simulink model "imageprocessing"  (R2024a)
settings: Solver=VariableStepAuto  StartTime=0.0  StopTime=10.0  RelTol=1e-3
undefined symbols (not defined in the file): CIRCLE_PTS, gray, ZEROS
libraries: visiontextngfix x1, parrotlib x1, simulink x1
settings Model: Creator=tejas  LastModifiedBy=tejas

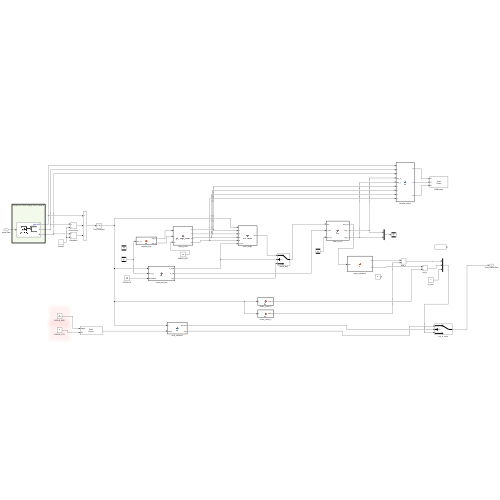
[thumbnail: Simulink's stored preview of the top-level diagram]
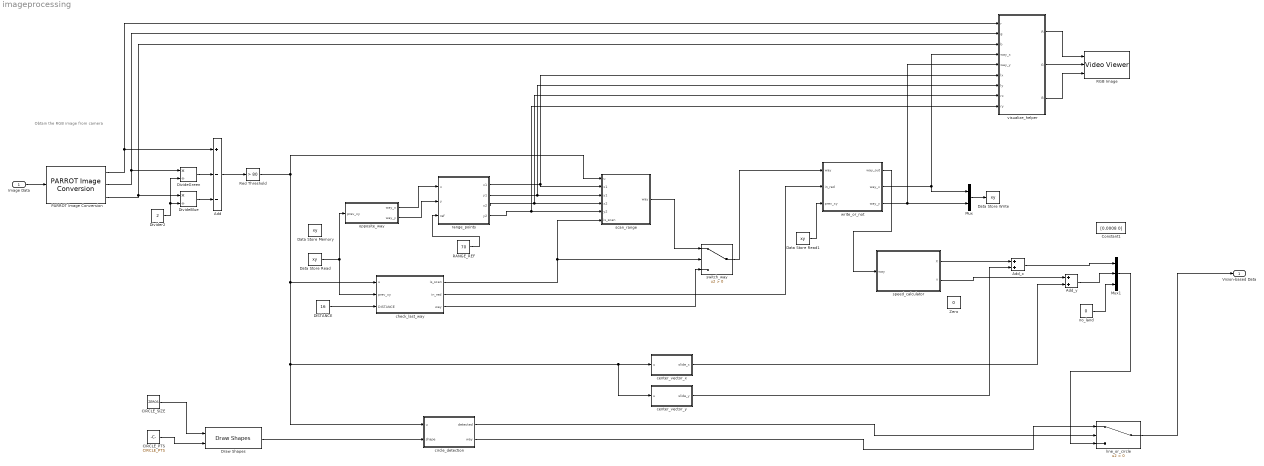
== system imageprocessing ==
  note: Obtain the RGB image from camera
  Image Data : Inport
  Add : Sum  Inputs=+--
  Add_x : Sum
  Add_y : Sum
  CIRCLE_PTS : Constant  Value=CIRCLE_PTS
  CIRCLE_SIZE : Constant  Value=ZEROS
  Constant1 : Constant  Value=[0.0008 0]
  DISTANCE : Constant  Value=16
  Data Store Memory : DataStoreMemory  DataStoreName=xy  ReadBeforeWriteMsg=warning  WriteAfterWriteMsg=warning  WriteAfterReadMsg=warning  InitialValue=[0 0]  ShowAdditionalParam=off
  Data Store Read : DataStoreRead  DataStoreName=xy  IndexOptions=Index vector (dialog)  Indices=1  OutputSizes=1
  Data Store Read1 : DataStoreRead  DataStoreName=xy  IndexOptions=Index vector (dialog)  Indices=1  OutputSizes=1
  Data Store Write : DataStoreWrite  DataStoreName=xy  IndexOptions=Index vector (dialog)  Indices=1  OutputSizes=1
  DivideBlue : Product  Inputs=*/
  DivideGreen : Product  Inputs=*/
  Divider2 : Constant  Value=2
  Draw Shapes : visiontextngfix/Draw Shapes  shape=Circles  fill=on  lineWidth=1  fillClrSource=Specify via dialog  display=White  intensity=200  color=[200 255 100]  opacity=1  viewport=Entire image  antialiasing=off  inType=Obsolete  imagePorts=One multidimensional signal  roundingMode=Floor  overflowMode=off  memoryMode=Specify word length  memoryWordLength=16  prodOutputMode=Binary point scaling  prodOutputWordLength=32  prodOutputFracLength=14  memoryFracLength=15
  Mux : Mux  Inputs=2
  Mux1 : Mux  Inputs=3
  PARROT Image Conversion : parrotlib/PARROT Image Conversion  ImageFormat=RGB  R=on  Y=on  G=on  U=on  B=on  V=on
  RANGE_REF : Constant  Value=70
  RGB Image : VideoViewer  imagePorts=separate color signals  colormapValue=gray(256)  FigPos=[2703.4 754 730.4 526.4]
  Red Threshold : simulink/Logic and Bit Operations/Compare To Constant  relop=>  const=80  OutDataTypeStr=boolean
  Zero : Constant  Value=0  OutDataTypeStr=Inherit: Inherit via back propagation
  center_vector_x : MATLAB Function  TreatAsAtomicUnit=on
  center_vector_y : MATLAB Function  TreatAsAtomicUnit=on
  check_last_way : MATLAB Function  TreatAsAtomicUnit=on
  circle_detection : MATLAB Function  TreatAsAtomicUnit=on
  line_or_circle : Switch  Criteria=u2 > Threshold  SaturateOnIntegerOverflow=off  InputSameDT=off
  no_land : Constant  Value=0
  opposite_way : MATLAB Function  TreatAsAtomicUnit=on
  range_points : MATLAB Function  TreatAsAtomicUnit=on
  scan_range : MATLAB Function  TreatAsAtomicUnit=on
  speed_calculator : MATLAB Function  TreatAsAtomicUnit=on
  switch_way : Switch  Criteria=u2 > Threshold  SaturateOnIntegerOverflow=off  InputSameDT=off
  visualize_helper : MATLAB Function  TreatAsAtomicUnit=on
  write_or_not : MATLAB Function  TreatAsAtomicUnit=on
  Vision-based Data : Outport  VectorParamsAs1DForOutWhenUnconnected=off
  wires:
  write_or_not/3(way_y) -> Mux/2, visualize_helper/5(way_y)
  write_or_not/2(way_x) -> Mux/1, visualize_helper/4(way_x)
  range_points/4(y2) -> scan_range/5(y2), visualize_helper/9(ry)
  speed_calculator/2(Y) -> Add_y/1
  opposite_way/2(way_y) -> range_points/2(y)
  visualize_helper/2(G) -> RGB Image/2
  Mux/1 -> Data Store Write/1
  PARROT Image Conversion/1 -> Add/1, visualize_helper/1(r)
  Image Data/1 -> PARROT Image Conversion/1
  range_points/1(x1) -> scan_range/2(x1), visualize_helper/6(lx)
  PARROT Image Conversion/3 -> visualize_helper/3(b), DivideBlue/1
  RANGE_REF/1 -> range_points/3(ref)
  write_or_not/1(way_out) -> speed_calculator/1(way)
  check_last_way/2(in_red) -> write_or_not/2(in_red)
  Data Store Read1/1 -> write_or_not/3(prev_xy)
  visualize_helper/1(R) -> RGB Image/1
  no_land/1 -> Mux1/3
  CIRCLE_PTS/1 -> Draw Shapes/2
  circle_detection/1(detected) -> line_or_circle/2
  DivideBlue/1 -> Add/3
  Data Store Read/1 -> opposite_way/1(prev_xy), check_last_way/2(prev_xy)
  center_vector_x/1(slide_x) -> Add_y/2
  PARROT Image Conversion/2 -> DivideGreen/1, visualize_helper/2(g)
  CIRCLE_SIZE/1 -> Draw Shapes/1
  check_last_way/1(is_scan) -> scan_range/6(is_scan), switch_way/2
  Add_x/1 -> Mux1/1
  circle_detection/2(way) -> line_or_circle/1
  speed_calculator/1(X) -> Add_x/1
  check_last_way/3(way) -> switch_way/3
  Add/1 -> Red Threshold/1
  range_points/3(x2) -> scan_range/4(x2), visualize_helper/8(rx)
  Divider2/1 -> DivideGreen/2, DivideBlue/2
  Red Threshold/1 -> circle_detection/1(u), center_vector_x/1(u), center_vector_y/1(u), check_last_way/1(u), scan_range/1(u)
  DivideGreen/1 -> Add/2
  switch_way/1 -> write_or_not/1(way)
  center_vector_y/1(slide_y) -> Add_x/2
  Add_y/1 -> Mux1/2
  opposite_way/1(way_x) -> range_points/1(x)
  scan_range/1(way) -> switch_way/1
  line_or_circle/1 -> Vision-based Data/1
  DISTANCE/1 -> check_last_way/3(DISTANCE)
  Mux1/1 -> line_or_circle/3
  Draw Shapes/1 -> circle_detection/2(shape)
  range_points/2(y1) -> scan_range/3(y1), visualize_helper/7(ly)
  visualize_helper/3(B) -> RGB Image/3

== matlab function imageprocessing/write_or_not ==
  data: way input; way_out output; in_red input; prev_xy input; way_x output; way_y output
function [way_out, way_x, way_y] = fcn(way, in_red, prev_xy)

x = way(1);
y = way(2);
speed = way(3);

if in_red
    X = x;   Y = y;
    way_x = x;  way_y = y;
else
    X = x;  Y = y; 
    way_x = prev_xy(1);  
    way_y = prev_xy(2);
end

way_out = [X Y speed];

%fprintf('X = %f | Y = %f\n', way_x, way_y);
end

== matlab function imageprocessing/speed_calculator ==
  data: way input; X output; Y output
function [X,Y] = fcn(way)

x = way(1);
y = way(2);
speed = way(3);

if speed == 100
    speed = 200;
elseif speed < 60
    speed = 60;
end


X = (60-x) / 10000000 * speed;
Y = (y-80) / 10000000 * speed;


%fprintf(' --- speed: %f | ', speed); fprintf('vectors: X=%.5f | Y=%.5f\n', X, Y);

end

== matlab function imageprocessing/opposite_way ==
  data: way_x output; prev_xy input; way_y output
function [way_x, way_y] = fcn(prev_xy)

    x = prev_xy(1);
    y = prev_xy(2);
    
    if x == 0 || y == 0
        way_x = 0;
        way_y = 0;
    else
        way_x = 60 + (60 - x) + 1;
        way_y = 80 + (80 - y) + 1;
    end

    %fprintf('opposite: %.0f %.0f -> %.0f %.0f\n', x, y, way_x, way_y);
end

== matlab function imageprocessing/center_vector_x ==
  data: u input; slide_x output
function slide_x = fcn(u)
c1 = 60; 
c2 = 80;
left_p = 0;
right_p = 0;
middle_point = u(c1, c2);
compare = ~middle_point;
for i = c2:-1:60 % <---  look left
    if u(c1, i) == compare
        left_p = i;
        break
    end
end
for i = c2:100 % --->   look right
    if u(c1, i) == compare
        right_p = i;
        break
    end
end

slide_x = 0;
if left_p ~= 0 && right_p ~= 0 % in line
    if middle_point == 1
        vr = right_p - c2;  % length right 
        vl = c2 - left_p;   % length left
        diff = vr-vl;
        slide_x = get_speed(diff) * 20;
    end
end
end

function T = get_speed(t)

if t > 0
    if t < 1
        T = 0.000001;
    elseif t < 5
        T = 0.000002;
    elseif t < 10
        T = 0.000003;
    elseif t < 15
        T = 0.000004;
    elseif t < 20
        T = 0.000005;
    else
        T = 0.000006;
    end
else
    if t < -20
        T = -0.000006;
    elseif t < -15
        T = -0.000005;
    elseif t < -10
        T = -0.000004;
    elseif t < -5
        T = -0.000003;
    elseif t < -1
        T = -0.000002;
    else
        T = -0.000001;
    end
end

end

== matlab function imageprocessing/range_points ==
  data: x input; x1 output; y input; ref input; y1 output; x2 output; y2 output
function [x1,y1, x2,y2] = get_range_points(x,y, ref)

% x1, y1 are left
% x2, y2 are right 
% according to center-to-edge vector.

W = edge_number(x,y);

if W == 1
    y1 = y - ref;
    if y1 < 1
        x1 = x - y1;
        y1 = 1;
    else
        x1 = x;
    end

    y2 = y + ref;
    if y2 > 160
        x2 = y2-160;
        y2 = 160;
    else
        x2 = x;
    end
elseif W == 2
    x1 = x + ref;
    if x1 > 120
        y1 = x1 - 120;
        x1 = 120;
    else
        y1 = y;
    end

    x2 = x - ref;
    if x2 < 1
        y2 = abs(x2) + 1;
        x2 = 1;
    else
        y2 = y;
    end
elseif W == 4
    x1 = x - ref;
    if x1 < 1
        y1 = 160 + x1;
        x1 = 1;
    else
        y1 = 160;
    end

    x2 = x + ref;
    if x2 > 120
        y2 = 160 - (x2 - 120);
        x2 = 120;
    else
        y2 = y;
    end
elseif W == 3
    y1 = y + ref;
    if y1 > 160
        x1 = 120 - (y1-160);
        y1 = 160;
    else
        x1 = x;
    end

    y2 = y - ref;
    if y2 < 1
        x2 = 120 + y2;
        y2 = 1;
    else
        x2 = x;
    end
else
    x1 = 1; y1 = 1;
    x2 = 1; y2 = 2;
end

%fprintf('range_points: %.0f-%.0f  to  %.0f-%.0f\n', x1,y1, x2,y2);

end

== matlab function imageprocessing/center_vector_y ==
  data: u input; slide_y output
function slide_y = fcn(u)
c1 = 60; 
c2 = 80;
up_p = 0;
down_p = 0;
middle_point = u(c1,c2);
compare = ~middle_point;
for i = c1:-1:40 % look up
    if u(i, c2) == compare
        up_p = i;
        break
    end
end
for i = c1:80 % look down
    if u(i, c2) == compare
        down_p = i;
        break
    end
end
slide_y = 0;
if up_p ~= 0 && down_p ~= 0  % in line
    if middle_point == 1
        vu = down_p - c1;  %length up
        vd = c1 - up_p;    %length down
        diff = vd-vu;
        
        slide_y = get_speed(diff) * 20;
    end
end

end
function T = get_speed(t)

if t > 0
    if t <= 1
        T = 0.000001;
    elseif t < 5
        T = 0.000002;
    elseif t < 10
        T = 0.000003;
    elseif t < 15
        T = 0.000005;
    elseif t < 20
        T = 0.000005;
    else
        T = 0.000005;
    end
else
    if t < -20
        T = -0.000005;
    elseif t < -15
        T = -0.000005;
    elseif t < -10
        T = -0.000004;
    elseif t <= -5
        T = -0.000003;
    elseif t < -1
        T = -0.000002;
    else
        T = -0.000001;
    end
end
end

== matlab function imageprocessing/scan_range ==
  data: way output; u input; x1 input; y1 input; x2 input; y2 input; is_scan input
function way  = scan_range(u, x1,y1, x2,y2, is_scan)

way_x = 1;
way_y = 2;
speed = 0;
in_red_line = u(60, 80);


persistent prev_endless_x;
persistent prev_endless_y;

if is_scan
    if in_red_line == 1  % ------ inside red-line ------
    
        t = 0;
        mx = 0;

        mx_endless_x = [0 0];
        mx_endless_y = [0 0];
        mx_t = [0 0];

        last_endless = false;
        index_of_endless = 0;
        
        w1 = edge_number(x1,y1);
        xi = x1;  yi = y1; k = 1;
        
        if w1 == 1 || w1 == 4
            k = -1;
        end
        
        
        while xi ~= x2 || yi ~= y2
            returned = line_drawer(60, 80, xi, yi, u, 0);

            if returned == 0 % if endless

                if last_endless == false
                    last_endless = true;
                    index_of_endless = index_of_endless + 1;
                end
                if index_of_endless > 2
                    break;
                end
                
                mx_endless_x(index_of_endless) = mx_endless_x(index_of_endless) + xi;
                mx_endless_y(index_of_endless) = mx_endless_y(index_of_endless) + yi;
                mx_t(index_of_endless) = mx_t(index_of_endless) + 1;

            else
                last_endless = false;
                if returned > mx
                    mx = returned;
                    way_x = xi; 
                    way_y = yi;
                    t = 1;
                end
            end

            % İteration
            temp_w = edge_number(xi, yi);
            if temp_w == 1 || temp_w == 3
                yi = yi + k;
            else
                xi = xi + k;
            end
            if xi < 1
                yi = 159; xi = 1; k = -1;
            elseif xi > 120
                xi = 120; yi = 2; k = 1;
            elseif yi < 1
                yi = 1; xi = 2; k = 1;
            elseif yi > 160
                yi = 160; xi = 119; k = -1;
            end
        end % while end


        if index_of_endless == 1 % ---------- 1 endless ------------
            %fprintf('only one endless!\n');
            way_x = mx_endless_x(1);
            way_y = mx_endless_y(1);
            t = mx_t(1);

            way_x = round(way_x/t);
            way_y = round(way_y/t);
            [way_x, way_y] = nearest_edge(way_x, way_y);

            prev_endless_x = 60 + (60 - way_x) + 1;
            prev_endless_y = 80 + (80 - way_y) + 1;

        elseif index_of_endless == 2 % ---------- 2 endless ------------
            
            if isempty(prev_endless_x)
                way_x = mx_endless_x(1);
                way_y = mx_endless_y(1);
                t = mx_t(1);
    
                way_x = round(way_x/t);
                way_y = round(way_y/t);
                [way_x, way_y] = nearest_edge(way_x, way_y);
    
                prev_endless_x = 60 + (60 - way_x) + 1;
                prev_endless_y = 80 + (80 - way_y) + 1;
            else
                mid_calculated = [0 0; 0 0];
                for i = 1:2
                    x = mx_endless_x(i);
                    y = mx_endless_y(i);
                    t = mx_t(i);

                    x = round(x/t);
                    y = round(y/t);
                    
                    [x,y] = nearest_edge(x, y);
                    
                    mid_calculated(i, 1) = x;
                    mid_calculated(i, 2) = y;
                end
                %fprintf('calculated = %.0f %.0f  | %.0f %.0f\n', ...
                %    mid_calculated(1,1), mid_calculated(1,2), ...
                %    mid_calculated(2,1), mid_calculated(2,2));

                diff_x1 = prev_endless_x-mid_calculated(1,1);
                diff_y1 = prev_endless_y-mid_calculated(1,2);
                diff_x2 = prev_endless_x-mid_calculated(2,1);
                diff_y2 = prev_endless_y-mid_calculated(2,2);
                diff1 = sqrt(diff_x1*diff_x1 + diff_y1*diff_y1);
                diff2 = sqrt(diff_x2*diff_x2 + diff_y2*diff_y2);

                if diff1 > diff2
                    way_x = mid_calculated(1,1);
                    way_y = mid_calculated(1,2);
                else
                    way_x = mid_calculated(2,1);
                    way_y = mid_calculated(2,2);
                end
                
                prev_endless_x = 60 + (60 - way_x) + 1;
                prev_endless_y = 80 + (80 - way_y) + 1;
                
            end
        else % ---------- NO endless ------------
            speed = mx;
        end

        

    else % ----------------- outside red line ----------------------
        x1 = 2; y1 = 1;
        x2 = 1; y2 = 1;
        
        ENDLESS = 100;
        mn = ENDLESS;
        w1 = edge_number(x1,y1);
        xi = x1;  yi = y1;  k = 1;
        if w1 == 1 || w1 == 4
            k = -1;
        end
        
        while xi ~= x2 || yi ~= y2
            returned = line_drawer(60, 80, xi, yi, u, 1);
    
            if returned > 0 && returned < mn
                mn = returned;
                way_x = xi;
                way_y = yi;
            end
    
            % İteration
            temp_w = edge_number(xi, yi);
            if temp_w == 1 || temp_w == 3
                yi = yi + k;
            else
                xi = xi + k;
            end
            if xi < 1
                yi = 159; xi = 1; k = -1;
            elseif xi > 120
                xi = 120; yi = 2; k = 1;
            elseif yi < 1
                yi = 1; xi = 2; k = 1;
            elseif yi > 160
                yi = 160; xi = 119; k = -1;
            end
        end % while
        
        speed = 100;
        if mn < 60
            speed = 60;
        end
    end % if redline end

end % is_scan

way = [way_x, way_y, speed];

end % function end

== matlab function imageprocessing/check_last_way ==
  data: u input; is_scan output; in_red output; prev_xy input; DISTANCE input; way output
function [is_scan, in_red, way]  = fcn(u, prev_xy, DISTANCE)

prev_x = prev_xy(1);
prev_y = prev_xy(2);

in_red = u(60, 80);
compare = ~in_red;

is_scan = 0;
way_x = 1;
way_y = 1;
speed = 0;

if prev_x == 0 || prev_y == 0
    is_scan = 1;
else 
    if u(prev_x, prev_y) == 1 

        % endless continue ------------------------------
        [ref_x, ref_y] = middle_point_of_endless_line(u, prev_x, prev_y);

        way_x = prev_x + ref_x;
        way_y = prev_y + ref_y;
        
        if way_y > 160
            if way_x == 120 
                way_x = 120 - mod(way_y, 160);
            elseif way_x == 1 
                way_x = mod(way_y, 160);
            end
            way_y = 160;
            
        elseif way_y < 1
            if way_x == 120 
                way_x = 120 - abs(way_y);
            elseif way_x == 1 
                way_x = abs(way_y); 
            end
            way_y = 1;
            
        elseif way_x < 1
            if way_y == 160
                way_y = 160 - abs(way_x);
            elseif way_y == 1
                way_y = abs(way_x);
            end
            way_x = 1;
            
        elseif way_x > 120
            if way_y == 160
                way_y = 160 - (way_x - 120);
            elseif way_y == 1
                way_y = way_x - 120;
            end
            way_x = 120;
        end

        %{
        if way_x < 1   way_x = 1;   end
        if way_x > 120 way_x = 120; end
        if way_y < 1   way_y = 1;   end
        if way_y > 160 way_y = 160; end
        %}
        speed = 100;

    else 
        
        % endless dissappeared ----------------------------
        if in_red
            distance = line_drawer(60, 80, prev_x, prev_y, u, compare);
            if distance < DISTANCE
                is_scan = 1;
                speed = 0;
            else
                speed = distance;
            end
            
            way_x = prev_x;
            way_y = prev_y;
        else
            is_scan = 1;
            way_x = prev_x;
            way_y = prev_y;
            speed = 40;
        end

    end
end
way = [way_x, way_y, speed];

end % func end



function [ref_x, ref_y] = middle_point_of_endless_line(u, way_x, way_y)

w = edge_number(way_x, way_y);

if w == 1 || w == 3

    % to right
    iter_y = way_y;
    iter_x = way_x;
    plus_or_minus = 1;
    x_or_y = 0; % 0:y   1:x
    distance = 0;

    while u(iter_x, iter_y) == 1
        if x_or_y == 0
            iter_y = iter_y + plus_or_minus;
        else
            iter_x = iter_x + plus_or_minus;
        end
        distance = distance + 1;
        
        if iter_y > 160
            iter_y = 160;
            x_or_y = 1;
            if iter_x == 120
                plus_or_minus = -1;
            elseif iter_x == 1
                plus_or_minus = 1;
            end
        end
        if iter_x < 1
            break;
        elseif iter_x > 120
            break;
        end
    end
    right = distance;

    % to left
    iter_y = way_y;
    iter_x = way_x;
    plus_or_minus = -1;
    x_or_y = 0; % 0:y   1:x
    distance = 0;
    
    while u(iter_x, iter_y) == 1
        if x_or_y == 0
            iter_y = iter_y + plus_or_minus;
        else
            iter_x = iter_x + plus_or_minus;
        end
        distance = distance + 1;

        if iter_y < 1
            iter_y = 1;
            x_or_y = 1;
            if iter_x == 120
                plus_or_minus = -1;
            elseif iter_x == 1
                plus_or_minus = 1;
            end
        end
        if iter_x < 1
            break
        elseif iter_x > 120
            break
        end
    end
    left = distance;
    
    
    ref_x = 0;
    diff = right - left;
    
    if abs(diff) >= 7 && abs(diff) < 25
        ref_y = round(diff/2);
    else
        ref_y = 0;
    end

else % ------------------------- 2 & 4 --------------------------
    % to up
    iter_x = way_x;
    iter_y = way_y;
    plus_or_minus = -1;
    x_or_y = 1; % 0:y   1:x
    distance = 0;
    while u(iter_x, iter_y) == 1
        if x_or_y == 0
            iter_y = iter_y + plus_or_minus;
        else
            iter_x = iter_x + plus_or_minus;
        end
        distance = distance + 1;

        if iter_x < 1
            iter_x = 1;
            x_or_y = 0;
            if iter_y == 1
                plus_or_minus = 1;
            elseif iter_y == 160
                plus_or_minus = -1;
            end
        end
        if iter_y > 160
            break
        elseif iter_y < 1
            break
        end
    end
    up = distance;

    % to down
    iter_x = way_x;
    iter_y = way_y;
    plus_or_minus = 1;
    x_or_y = 1; % 0:y   1:x
    distance = 0;
    while u(iter_x, iter_y) == 1
        if x_or_y == 0
            iter_y = iter_y + plus_or_minus;
        else
            iter_x = iter_x + plus_or_minus;
        end
        distance = distance + 1;
        if iter_x > 120
            x_or_y = 0;
            iter_x = 120;
            if iter_y == 1
                plus_or_minus = 1;
            elseif iter_y == 160
                plus_or_minus = -1;
            end
        end
        if iter_y > 160
            break;
        elseif iter_y < 1
            break;
        end
    end
    down = distance;

    diff = down - up;

    ref_y = 0;
    if abs(diff) >= 7 && abs(diff) < 25
        ref_x = round(diff/2);
    else
        ref_x = 0;
    end
end

end

== matlab function imageprocessing/circle_detection ==
  data: u input; detected output; shape input; way output
function [detected, way] = fcn(u, shape)

persistent landing;
if isempty(landing)
    landing = 0;
end

detected = 0;
way = [0 0 0];
land = 0;

if landing == 1
    way = [0 0 1];
    detected = 1;

else
    [total_pixel, cord_x, cord_y] = detect_circle(u, shape);
    
    if total_pixel >= 1350
        detected = 1;
        center_x = cord_x + 19;
        center_y = cord_y + 19;
    
        if center_x > 120
            center_x = 120;
        end
        if center_y > 160
            center_y = 160;
        end
        
        
        dif_x = round(60 - center_x);
        dif_y = round(center_y - 80);
        
        dist = sqrt(dif_x * dif_x + dif_y * dif_y);
    
        fprintf(' #### CIRCLE - centers: %3.1f %3.1f | dist: %3.1f\n', ...
            center_x, center_y, dist);
    
        if dist < 15
            land = 1;
            landing = 1;
        end
        way_x = dif_x / 130000;
        way_y = dif_y / 130000;
        way = [way_x way_y land];
    end

end

end

function [total_pixel, cord_x, cord_y] = detect_circle(u, shape)

%  total_pixel: sum of number of pixel
%       cord_x: row coordinate of u
%       cord_y: column coordinate of u

[circle_size_x, circle_size_y] = size(shape);
R = 120;  C = 160;

total_pixel = 0;
cord_x = 0;
cord_y = 0;

for i = 1:(R - circle_size_x)
    for j = 1:(C - circle_size_y)
        section = u(i:i+circle_size_x-1, j:j+circle_size_y-1);
        result = sum(~xor(section, shape), 'all');
        if result > total_pixel
            total_pixel = result;
            cord_x = i;
            cord_y = j;
        end
    end

end
end

== matlab function imageprocessing/visualize_helper ==
  data: r input; R output; g input; b input; way_x input; way_y input; G output; B output; lx input; ly input; rx input; ry input
function [R,G,B] = fcn(r,g,b, way_x, way_y,  lx,ly, rx,ry)

% completely unnecessary block for algorithm, just for visualize

r(60,80) = 255; g(60,80) = 255; b(60,80) = 255;

if way_x >= 1 && way_y >= 1 && way_x <= 120 && way_y <= 160


% -----------------------------------------------
    x1 = 60; y1 = 80;  x2 = way_x;   y2 = way_y;
    swapepd = 0;
    if abs(y2 - y1) > abs(x2 - x1)
        %disp('[swapped] dy bigger')
        swapepd = 1;
        [x1,y1] = deal(y1,x1);
        [x2,y2] = deal(y2,x2);
        xk = 1; yk = 1;
        if (x2 < x1) xk = -1; end
        if (y2 < y1) yk = -1; end
    else
        xk = -1; yk = -1;
        if (x2 > x1) xk = 1; end
        if (y2 > y1) yk = 1; end

    end
    dy = abs(y2-y1);
    dx = abs(x2-x1);
    % --------------------------------------
    m = 2 * dy;
    slope_error = m - 2*dx;
  
    y = y1;
    for x = x1:xk:x2
        if swapepd == 1
            r(y,x) = 255; g(y,x) = 255; b(y,x) = 255;
        else
            r(x,y) = 255; g(x,y) = 255; b(x,y) = 255;
        end
        
   
        slope_error = slope_error + m;
        if (slope_error > 0)
            y = y + yk;
            slope_error = slope_error - 2 * dx;
        end
    end
end




% --------------------------------------------
x1 = 60; y1 = 80; x2 = lx; y2 = ly;
    swapepd = 0;
    if abs(y2 - y1) > abs(x2 - x1)
        %disp('[swapped] dy bigger')
        swapepd = 1;
        [x1,y1] = deal(y1,x1);
        [x2,y2] = deal(y2,x2);
        xk = 1; yk = 1;
        if (x2 < x1) xk = -1; end
        if (y2 < y1) yk = -1; end
    else
        xk = -1; yk = -1;
        if (x2 > x1) xk = 1; end
        if (y2 > y1) yk = 1; end

    end
    dy = abs(y2-y1);
    dx = abs(x2-x1);
    % --------------------------------------
    m = 2 * dy;
    slope_error = m - 2*dx;
  
    y = y1;
    for x = x1:xk:x2
        if swapepd == 1
            g(y,x) = 255;
        else
            g(x,y) = 255;
        end
        
   
        slope_error = slope_error + m;
        if (slope_error > 0)
            y = y + yk;
            slope_error = slope_error - 2 * dx;
        end
    end
% -----------------------------------------

    x1 = 60; y1 = 80; x2 = rx; y2 = ry;
    swapepd = 0;
    if abs(y2 - y1) >= abs(x2 - x1)
        %disp('[swapped] dy bigger')
        swapepd = 1;
        [x1,y1] = deal(y1,x1);
        [x2,y2] = deal(y2,x2);
        xk = 1; yk = 1;
        if (x2 < x1) xk = -1; end
        if (y2 < y1) yk = -1; end
    else
        xk = -1; yk = -1;
        if (x2 > x1) xk = 1; end
        if (y2 > y1) yk = 1; end

    end
    dy = abs(y2-y1);
    dx = abs(x2-x1);
    % --------------------------------------
    m = 2 * dy;
    slope_error = m - 2*dx;
  
    y = y1;
    for x = x1:xk:x2
        if swapepd == 1
            if x <1 break; end
            g(y,x) = 255;
        else
            g(x,y) = 255;
        end
        
   
        slope_error = slope_error + m;
        if (slope_error > 0)
            y = y + yk;
            slope_error = slope_error - 2 * dx;
        end
    end

b(40:80, 60:90) = 200;
R = r;
G = g;
B = b;
end
